simulink model "stab_mez_cyklu"  (R2018a)
settings: Solver=FixedStepAuto  StartTime=0.0  StopTime=150  FixedStep=0.01  RelTol=1e-3
libraries: simulink x1
settings Model: Creator=vejvarm  LastModifiedBy=vejvarm

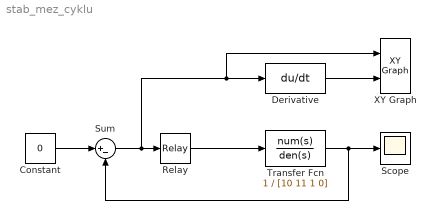
== system stab_mez_cyklu ==
  Constant : Constant  Value=0
  Derivative : Derivative
  Relay : Relay  OnSwitchValue=0  OffSwitchValue=0  OffOutputValue=-1
  Scope : Scope
  Sum : Sum  Inputs=|+-
  Transfer Fcn : TransferFcn  Numerator=1  Denominator=[10 11 1 0]
  XY Graph : simulink/Sinks/XY Graph  xmin=-1.5  xmax=1.5  ymin=-0.5  ymax=0.5  st=-1
  wires:
  Relay/1 -> Transfer Fcn/1
  Sum/1 -> XY Graph/1, Derivative/1, Relay/1
  Transfer Fcn/1 -> Scope/1, Sum/2
  Constant/1 -> Sum/1
  Derivative/1 -> XY Graph/2
